simulink model "Lab6_4"  (R2021a)
settings: Solver=VariableStepAuto  StartTime=0.0  StopTime=.07  RelTol=1e-3  EnableMultiTasking=on
libraries: spsIGBTDiodeLib x24, spsDCVoltageSourceLib x6, spsVoltageMeasurementLib x4, spsCurrentMeasurementLib x3, spsSeriesRLCBranchLib x3, spsTriangleGeneratorLib x1, spspowerguiLib x1
settings Model: Creator=usee  LastModifiedBy=User
settings SolverCC: AlgebraicLoopSolver=TrustRegion
settings DataIOCC: ReturnWorkspaceOutputs=off
settings OptimizationCC: LifeSpan=inf
settings DebuggingCC: SFUnexpectedBacktrackingDiag=warning  SFNoUnconditionalDefaultTransitionDiag=warning  SFMachineParentedDataDiag=warning  ArithmeticOperatorsInVariantConditions=warning
settings SFSimCC: SimUseLocalCustomCode=off  CustomCodeUndefinedFunction=UseInterfaceOnly
settings RTWCC: RTWUseLocalCustomCode=off
settings CodeAppCC: StateflowObjectComments=on
settings GRTTargetCC: TargetLangStandard=C89/C90 (ANSI)
settings ConfigComp: CovMetricSettings=dw  CovSaveCumulativeToWorkspaceVar=on  CovSaveSingleToWorkspaceVar=on  CovExternalEMLEnable=off
settings SimscapeCC: SimscapeNormalizeSystem=off

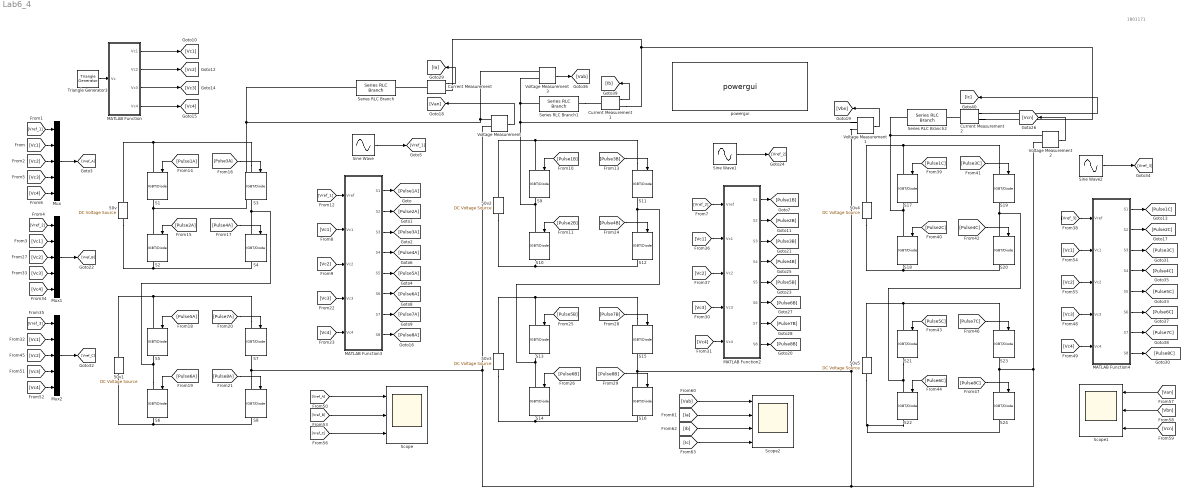
== system Lab6_4 ==
  note: 1801171
  50v{,1..5} (6 alike) : spsDCVoltageSourceLib/DC Voltage Source  Amplitude=50  Measurements=None
  Current Measurement : spsCurrentMeasurementLib/Current Measurement  PhasorSimulation=off  OutputType=Complex  PSBequivalent=0
  Current Measurement1 : spsCurrentMeasurementLib/Current Measurement  PhasorSimulation=off  OutputType=Complex  PSBequivalent=0
  Current Measurement2 : spsCurrentMeasurementLib/Current Measurement  PhasorSimulation=off  OutputType=Complex  PSBequivalent=0
  MATLAB Function : MATLAB Function  TreatAsAtomicUnit=on
  MATLAB Function2 : MATLAB Function  TreatAsAtomicUnit=on
  MATLAB Function3 : MATLAB Function  TreatAsAtomicUnit=on
  MATLAB Function4 : MATLAB Function  TreatAsAtomicUnit=on
  Mux : Mux  Inputs=5
  Mux1 : Mux  Inputs=5
  Mux2 : Mux  Inputs=5
  S{1..24} (24 alike) : spsIGBTDiodeLib/IGBT//Diode  Ron=1e-3  Rs=1e5  Cs=inf  Measurements=on
  Scope : Scope  NumInputPorts=3
  Scope1 : Scope  NumInputPorts=3
  Scope2 : Scope  NumInputPorts=4
  Series RLC Branch : spsSeriesRLCBranchLib/Series RLC Branch  LConnTagsString=__new0  RConnTagsString=__new0  BranchType=RL  Resistance=5  Inductance=100e-3  SetiL0=off  InitialCurrent=0  Capacitance=1e-6  Setx0=off  InitialVoltage=0  Measurements=None
  Series RLC Branch1 : spsSeriesRLCBranchLib/Series RLC Branch  LConnTagsString=__new0  RConnTagsString=__new0  BranchType=RL  Resistance=5  Inductance=100e-3  SetiL0=off  InitialCurrent=0  Capacitance=1e-6  Setx0=off  InitialVoltage=0  Measurements=None
  Series RLC Branch2 : spsSeriesRLCBranchLib/Series RLC Branch  LConnTagsString=__new0  RConnTagsString=__new0  BranchType=RL  Resistance=5  Inductance=100e-3  SetiL0=off  InitialCurrent=0  Capacitance=1e-6  Setx0=off  InitialVoltage=0  Measurements=None
  Sine Wave : Sin  Frequency=2*pi*50  SampleTime=0
  Sine Wave1 : Sin  Frequency=2*pi*50  Phase=120*pi/180  SampleTime=0
  Sine Wave2 : Sin  Frequency=2*pi*50  Phase=240*pi/180  SampleTime=0
  Triangle Generator3 : spsTriangleGeneratorLib/Triangle Generator  Freq=1000  Phase=0  Ts=0
  Voltage Measurement{,1..3} (4 alike) : spsVoltageMeasurementLib/Voltage Measurement  PhasorSimulation=off  OutputType=Complex  PSBequivalent=0
  powergui : spspowerguiLib/powergui  Priority=1  SimulationMode=Discrete  SampleTime=50e-6  frequency=60  Iterations=50  frequencyindice=0  Pbase=100e6  ErrMax=1e-4  UnitsV=kV  UnitsW=MW  buscounter=0  FunctionMessages=off  echomessages=off  EnableUseOfTLC=off  CurrentSourceSwitches=off  DisableSnubberDevices=off  DisableRonSwitches=off  DisableVfSwitches=off  DisplayEquations=off  AutomaticDiscreteSolvers=off  SolverType=Tustin/Backward Euler (TBE)  Interpol=off  ExternalGateDelay=off  methode=off  Ts=10  x0status=blocks  SPID=off  SwTol=0  HookPort=off  NonlinearTolerance=1e-4  nMaxIteration=100  ContinueOnMaxIteration=off  RestoreLinks=warning  ResistiveCurrentMeasurement=off  Frange=[0:2:500]  Ylog=off  Xlog=on  ShowGrid=off  save=off  variable=ZData  structure=I  ZoomFFT=on  StartTime=0.2  cycles=5  DisplayStyle=2  fundamental=50  FreqAxis=off  MaxFrequency=1000  frequencyindicesteady=1  RmsSteady=1  display=off
  wires:
  [Vc1] -> MATLAB Function3/2(Vc1)
  MATLAB Function3/6(S6) -> [Pulse6A]
  MATLAB Function3/5(S5) -> [Pulse5A]
  [Pulse1A] -> S1/1
  [Pulse2A] -> S2/1
  [Pulse5A] -> S5/1
  [Pulse7A] -> S7/1
  [Pulse6A] -> S6/1
  [Pulse8A] -> S8/1
  [Pulse4A] -> S4/1
  MATLAB Function3/8(S8) -> [Pulse8A]
  [Vc3] -> MATLAB Function3/4(Vc3)
  MATLAB Function3/2(S2) -> [Pulse2A]
  [Vc4] -> MATLAB Function3/5(Vc4)
  MATLAB Function3/1(S1) -> [Pulse1A]
  MATLAB Function3/3(S3) -> [Pulse3A]
  [Pulse3A] -> S3/1
  [Vref_1] -> MATLAB Function3/1(Vref)
  MATLAB Function3/7(S7) -> [Pulse7A]
  MATLAB Function3/4(S4) -> [Pulse4A]
  [Vc2] -> MATLAB Function3/3(Vc2)
  [Vc2] -> MATLAB Function2/3(Vc2)
  MATLAB Function2/4(S4) -> [Pulse4B]
  MATLAB Function2/7(S7) -> [Pulse7B]
  [Vref_2] -> MATLAB Function2/1(Vref)
  [Pulse3B] -> S11/1
  MATLAB Function2/3(S3) -> [Pulse3B]
  MATLAB Function2/1(S1) -> [Pulse1B]
  [Vc4] -> MATLAB Function2/5(Vc4)
  MATLAB Function2/2(S2) -> [Pulse2B]
  [Vc3] -> MATLAB Function2/4(Vc3)
  MATLAB Function2/8(S8) -> [Pulse8B]
  [Pulse4B] -> S12/1
  [Pulse8B] -> S16/1
  [Pulse6B] -> S14/1
  [Pulse7B] -> S15/1
  [Pulse5B] -> S13/1
  [Pulse2B] -> S10/1
  [Pulse1B] -> S9/1
  MATLAB Function2/5(S5) -> [Pulse5B]
  MATLAB Function2/6(S6) -> [Pulse6B]
  [Vc1] -> MATLAB Function2/2(Vc1)
  [Vc1] -> MATLAB Function4/2(Vc1)
  MATLAB Function4/6(S6) -> [Pulse6C]
  MATLAB Function4/5(S5) -> [Pulse5C]
  [Pulse1C] -> S17/1
  [Pulse2C] -> S18/1
  [Pulse5C] -> S21/1
  [Pulse7C] -> S23/1
  [Pulse6C] -> S22/1
  [Pulse8C] -> S24/1
  [Pulse4C] -> S20/1
  MATLAB Function4/8(S8) -> [Pulse8C]
  [Vc3] -> MATLAB Function4/4(Vc3)
  MATLAB Function4/2(S2) -> [Pulse2C]
  [Vc4] -> MATLAB Function4/5(Vc4)
  MATLAB Function4/1(S1) -> [Pulse1C]
  MATLAB Function4/3(S3) -> [Pulse3C]
  [Pulse3C] -> S19/1
  [Vref_3] -> MATLAB Function4/1(Vref)
  MATLAB Function4/7(S7) -> [Pulse7C]
  MATLAB Function4/4(S4) -> [Pulse4C]
  [Vc2] -> MATLAB Function4/3(Vc2)
  Voltage Measurement/1 -> [Van]
  Voltage Measurement1/1 -> [Vbn]
  Voltage Measurement2/1 -> [Vcn]
  Current Measurement/1 -> [Ia]
  Triangle Generator3/1 -> MATLAB Function/1(Vc)
  MATLAB Function/4(Vc4) -> [Vc4]
  MATLAB Function/3(Vc3) -> [Vc3]
  MATLAB Function/2(Vc2) -> [Vc2]
  MATLAB Function/1(Vc1) -> [Vc1]
  Sine Wave/1 -> [Vref_1]
  Mux/1 -> [Vref_A]
  [Vc4] -> Mux/5
  [Vc2] -> Mux/3
  [Vref_1] -> Mux/1
  [Vc1] -> Mux/2
  [Vc3] -> Mux/4
  [Vc3] -> Mux1/4
  [Vc1] -> Mux1/2
  [Vref_2] -> Mux1/1
  [Vc2] -> Mux1/3
  [Vc4] -> Mux1/5
  Mux1/1 -> [Vref_B]
  Sine Wave1/1 -> [Vref_2]
  Mux2/1 -> [Vref_C]
  [Vc4] -> Mux2/5
  [Vc2] -> Mux2/3
  [Vref_3] -> Mux2/1
  [Vc1] -> Mux2/2
  [Vc3] -> Mux2/4
  Sine Wave2/1 -> [Vref_3]
  Voltage Measurement3/1 -> [Vab]
  [Vref_A] -> Scope/1
  [Vref_B] -> Scope/2
  [Vref_C] -> Scope/3
  [Van] -> Scope1/1
  [Vbn] -> Scope1/2
  [Vcn] -> Scope1/3
  [Vab] -> Scope2/1
  [Ia] -> Scope2/2
  Current Measurement1/1 -> [Ib]
  Current Measurement2/1 -> [Ic]
  [Ib] -> Scope2/3
  [Ic] -> Scope2/4
  connections:
  S6/RConn1 -- 50v1/LConn1 -- S8/RConn1
  S7/LConn1 -- 50v1/RConn1 -- S5/LConn1
  S3/LConn1 -- 50v/RConn1 -- S1/LConn1
  S6/LConn1 -- S5/RConn1 -- S4/LConn1 -- S3/RConn1
  S4/RConn1 -- 50v/LConn1 -- S2/RConn1
  S12/RConn1 -- S10/RConn1 -- 50v2/LConn1
  S12/LConn1 -- S13/RConn1 -- S14/LConn1 -- S11/RConn1
  S11/LConn1 -- 50v2/RConn1 -- S9/LConn1
  S15/LConn1 -- 50v3/RConn1 -- S13/LConn1
  S16/RConn1 -- 50v3/LConn1 -- S14/RConn1
  S22/RConn1 -- 50v5/LConn1 -- S24/RConn1
  S1/RConn1 -- Series RLC Branch/LConn1 -- Voltage Measurement3/LConn1 -- Voltage Measurement/LConn1 -- S2/LConn1
  S21/LConn1 -- 50v5/RConn1 -- S23/LConn1
  S19/LConn1 -- 50v4/RConn1 -- S17/LConn1
  S21/RConn1 -- S20/LConn1 -- S19/RConn1 -- S22/LConn1
  S20/RConn1 -- 50v4/LConn1 -- S18/RConn1
  S8/LConn1 -- Voltage Measurement/LConn2 -- S15/RConn1 -- S16/LConn1 -- Voltage Measurement1/LConn2 -- Voltage Measurement2/LConn2 -- S24/LConn1 -- S23/RConn1 -- S7/RConn1
  S17/RConn1 -- Voltage Measurement2/LConn1 -- Series RLC Branch2/LConn1 -- S18/LConn1
  Voltage Measurement1/LConn1 -- Series RLC Branch1/LConn1 -- Voltage Measurement3/LConn2 -- S9/RConn1 -- S10/LConn1
  Current Measurement1/RConn1 -- Current Measurement/RConn1 -- Current Measurement2/RConn1
  Current Measurement/LConn1 -- Series RLC Branch/RConn1
  Series RLC Branch1/RConn1 -- Current Measurement1/LConn1
  Current Measurement2/LConn1 -- Series RLC Branch2/RConn1

== matlab function Lab6_4/MATLAB Function ==
  data: Vc input; Vc1 output; Vc2 output; Vc3 output; Vc4 output
function [Vc1,Vc2,Vc3,Vc4] = fcn(Vc)

Vc1 = (Vc+1)/4;
Vc2=Vc1+0.5;
Vc3= (Vc+1)/(-4);
Vc4=Vc3-0.5;

end

== matlab function Lab6_4/MATLAB Function3 ==
  data: Vref input; S1 output; Vc1 input; Vc2 input; S2 output; S3 output; S4 output; Vc3 input; Vc4 input; S5 output; S6 output; S7 output; S8 output
function [S1,S2,S3,S4,S5,S6,S7,S8]  = fcn(Vref,Vc1,Vc2,Vc3,Vc4)
 
if Vref >0
    if Vref>=0 && Vref<=0.5
        if Vref>=Vc1
            S1 =1;     S2 =0;     S3 =0;     S4 =1;     S5 =1;    S6 =0;     S7 =1;     S8 =0;
        else
            S1 =1;     S2 =0;     S3 =1;     S4 =0;     S5 =1;    S6 =0;     S7 =1;     S8 =0;
        end
        
    else
        if Vref>=Vc2
            S1 =1;     S2 =0;     S3 =0;     S4 =1;     S5 =1;     S6 =0;     S7 =0;     S8 =1;
        else
            S1 =1;     S2 =0;     S3 =0;     S4 =1;     S5 =1;     S6 =0;     S7 =1;     S8 =0;
        end
    end        
    
else
    if Vref<=0 && Vref>=-0.5
        if Vref<=Vc3
            S1 =0;     S2 =1;     S3 =1;     S4 =0;     S5 =1;     S6 =0;     S7 =1;     S8 =0;
        else
            S1 =0;     S2 =1;     S3 =0;     S4 =1;     S5 =0;     S6 =1;     S7 =0;     S8 =1;
        end
         
    else
        if Vref<=Vc4
            S1 =0;     S2 =1;     S3 =1;     S4 =0;     S5 =0;     S6 =1;     S7 =1;     S8 =0;
        else
            S1 =0;     S2 =1;     S3 =1;     S4 =0;     S5 =1;     S6 =0;     S7 =1;     S8 =0;
        end
    end      
end    
end

== matlab function Lab6_4/MATLAB Function2 ==
  data: Vref input; S1 output; Vc1 input; Vc2 input; S2 output; S3 output; S4 output; Vc3 input; Vc4 input; S5 output; S6 output; S7 output; S8 output
function [S1,S2,S3,S4,S5,S6,S7,S8]  = fcn(Vref,Vc1,Vc2,Vc3,Vc4)
 
if Vref >0
    if Vref>=0 && Vref<=0.5
        if Vref>=Vc1
            S1 =1;     S2 =0;     S3 =0;     S4 =1;     S5 =1;    S6 =0;     S7 =1;     S8 =0;
        else
            S1 =1;     S2 =0;     S3 =1;     S4 =0;     S5 =1;    S6 =0;     S7 =1;     S8 =0;
        end
        
    else
        if Vref>=Vc2
            S1 =1;     S2 =0;     S3 =0;     S4 =1;     S5 =1;     S6 =0;     S7 =0;     S8 =1;
        else
            S1 =1;     S2 =0;     S3 =0;     S4 =1;     S5 =1;     S6 =0;     S7 =1;     S8 =0;
        end
    end        
    
else
    if Vref<=0 && Vref>=-0.5
        if Vref<=Vc3
            S1 =0;     S2 =1;     S3 =1;     S4 =0;     S5 =1;     S6 =0;     S7 =1;     S8 =0;
        else
            S1 =0;     S2 =1;     S3 =0;     S4 =1;     S5 =0;     S6 =1;     S7 =0;     S8 =1;
        end
         
    else
        if Vref<=Vc4
            S1 =0;     S2 =1;     S3 =1;     S4 =0;     S5 =0;     S6 =1;     S7 =1;     S8 =0;
        else
            S1 =0;     S2 =1;     S3 =1;     S4 =0;     S5 =1;     S6 =0;     S7 =1;     S8 =0;
        end
    end      
end    
end

== matlab function Lab6_4/MATLAB Function4 ==
  data: Vref input; S1 output; Vc1 input; Vc2 input; S2 output; S3 output; S4 output; Vc3 input; Vc4 input; S5 output; S6 output; S7 output; S8 output
function [S1,S2,S3,S4,S5,S6,S7,S8]  = fcn(Vref,Vc1,Vc2,Vc3,Vc4)
 
if Vref >0
    if Vref>=0 && Vref<=0.5
        if Vref>=Vc1
            S1 =1;     S2 =0;     S3 =0;     S4 =1;     S5 =1;    S6 =0;     S7 =1;     S8 =0;
        else
            S1 =1;     S2 =0;     S3 =1;     S4 =0;     S5 =1;    S6 =0;     S7 =1;     S8 =0;
        end
        
    else
        if Vref>=Vc2
            S1 =1;     S2 =0;     S3 =0;     S4 =1;     S5 =1;     S6 =0;     S7 =0;     S8 =1;
        else
            S1 =1;     S2 =0;     S3 =0;     S4 =1;     S5 =1;     S6 =0;     S7 =1;     S8 =0;
        end
    end        
    
else
    if Vref<=0 && Vref>=-0.5
        if Vref<=Vc3
            S1 =0;     S2 =1;     S3 =1;     S4 =0;     S5 =1;     S6 =0;     S7 =1;     S8 =0;
        else
            S1 =0;     S2 =1;     S3 =0;     S4 =1;     S5 =0;     S6 =1;     S7 =0;     S8 =1;
        end
         
    else
        if Vref<=Vc4
            S1 =0;     S2 =1;     S3 =1;     S4 =0;     S5 =0;     S6 =1;     S7 =1;     S8 =0;
        else
            S1 =0;     S2 =1;     S3 =1;     S4 =0;     S5 =1;     S6 =0;     S7 =1;     S8 =0;
        end
    end      
end    
end
